simulink library "PIDController_ul"  (R2018b)
settings: Solver=VariableStepAuto  StartTime=0.0  StopTime=10.0  RelTol=1e-3
undefined symbols (not defined in the file): kd, ki, kp, tau
settings Model: Creator=mcobb  LastModifiedBy=mcobb

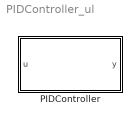
== system PIDController_ul ==
  PIDController : Subsystem  mask{kp=kp, ki=ki, kd=kd, Value=tau}
      mask prompts: kp "Proportional Gain, kp"; ki "Integral Gain, ki"; kd "Derivative Gain, kd"; Value "Time Constant, s"
      mask TypeOptions kp: kp/Gain
      mask TypeOptions ki: ki/Gain
      mask TypeOptions kd: kd/Gain
      mask TypeOptions Value: tau/Value

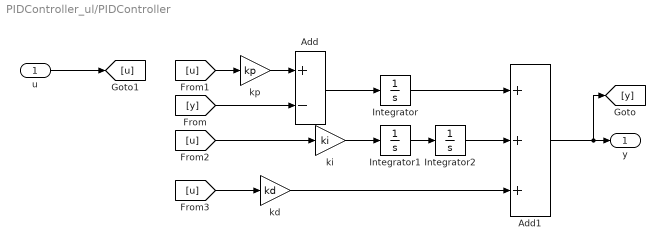
== system PIDController_ul/PIDController ==
  u : Inport  PortDimensions=1
  Add : Sum  Inputs=+-
  Add1 : Sum  Inputs=+++
  Integrator : Integrator
  Integrator1 : Integrator
  Integrator2 : Integrator
  kd : Gain  Gain=kd
  ki : Gain  Gain=ki
  kp : Gain  Gain=kp
  y : Outport  PortDimensions=1
  wires:
  u/1 -> [u]
  kp/1 -> Add/1
  [y] -> Add/2
  Add/1 -> Integrator/1
  [u] -> kp/1
  Integrator1/1 -> Integrator2/1
  ki/1 -> Integrator1/1
  [u] -> ki/1
  [u] -> kd/1
  Integrator2/1 -> Add1/2
  Integrator/1 -> Add1/1
  kd/1 -> Add1/3
  Add1/1 -> [y], y/1
